simulink model "EPD_5_gen_with_limits_dell_p_values"  (R2021b)
settings: Solver=VariableStepAuto  StartTime=0.0  StopTime=50  RelTol=1e-3
settings Model: Creator=vijay  LastModifiedBy=vijay

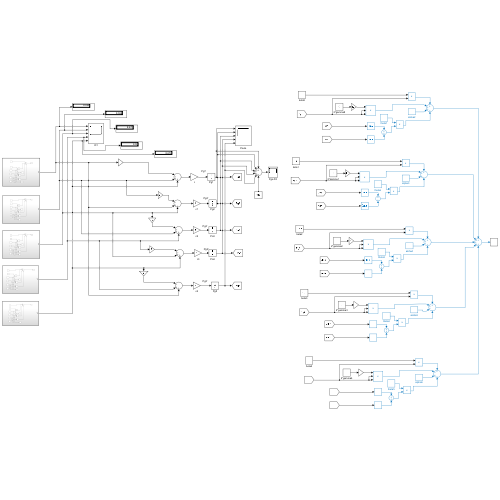
[thumbnail: Simulink's stored preview of the top-level diagram]
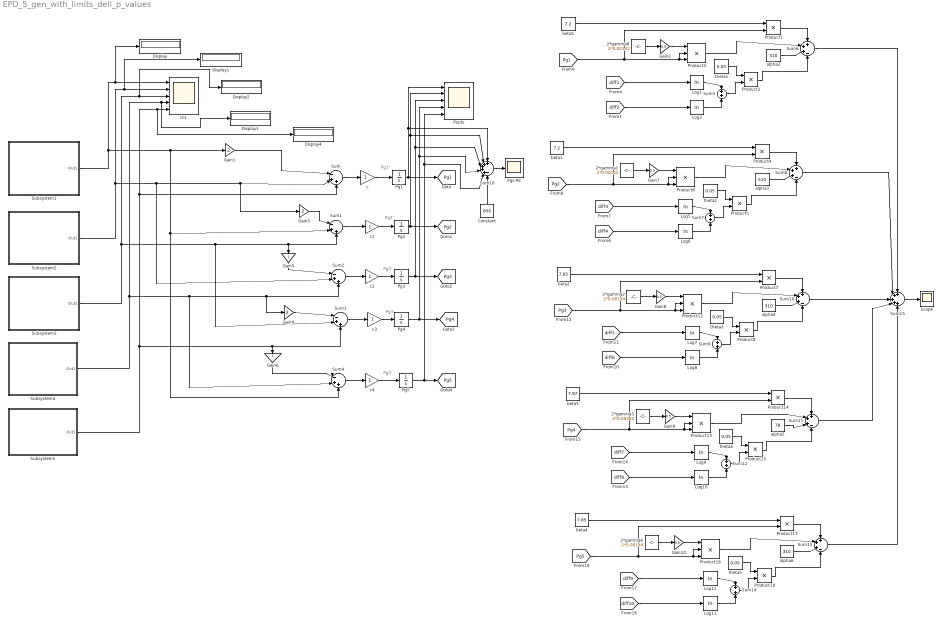
== system EPD_5_gen_with_limits_dell_p_values ==
  note: Pg3'
  note: Pg2'
  note: Pg1'
  note: Pg3'
  note: Pg3'
  2*gamma1 : Constant  Value=2*0.00142
  2*gamma2 : Constant  Value=2*0.00194
  2*gamma3 : Constant  Value=2*0.00482
  2*gamma4 : Constant  Value=2*0.00194
  2*gamma8 : Constant  Value=2*0.00142
  Constant : Constant  Value=850
  Display{,1..4} (5 alike) : Display
  Gain{1,3..6} (5 alike) : Gain  Gain=2
  Gain{2,7..10} (5 alike) : Gain  Gain=0.5
  IC1 : Scope  NumInputPorts=5
  Log{1,3,5..12} (10 alike) : Math  Operator=log  SignedPower=on  SaturateOnIntegerOverflow=on
  Pg1 : Integrator  InitialCondition=260
  Pg2 : Integrator  InitialCondition=260
  Pg3 : Integrator  InitialCondition=220
  Pg4 : Integrator  InitialCondition=170
  Pg5 : Integrator  InitialCondition=220
  Pgs-Pd : Scope
  Pouts : Scope  NumInputPorts=5
  Product{1..2,4..5,7..8,14..15,17..18} (10 alike) : Product
  Product{3,6,12..13,16} (5 alike) : Product  Inputs=3
  Scope : Scope
  Subsystem1 : Subsystem
  Subsystem2 : Subsystem
  Subsystem3 : Subsystem
  Subsystem4 : Subsystem
  Subsystem5 : Subsystem
  Sum{,1..4} (5 alike) : Sum  Inputs=|-++
  Sum{6,8,10..11,13} (5 alike) : Sum  Inputs=+++-
  Sum{5,7,9,12,14} (5 alike) : Sum
  Sum15 : Sum  Inputs=+++++
  Sum16 : Sum  Inputs=+++++-
  alpha2 : Constant  Value=510
  alpha3 : Constant  Value=510
  alpha4 : Constant  Value=310
  alpha5 : Constant  Value=78
  alpha6 : Constant  Value=310
  beta1 : Constant  Value=7.2
  beta2 : Constant  Value=7.85
  beta3 : Constant  Value=7.97
  beta4 : Constant  Value=7.85
  beta5 : Constant  Value=7.2
  c{,1..4} (5 alike) : Gain
  theta{1..5} (5 alike) : Constant  Value=0.05
  tag scope: Pg1=global, Pg2=global, Pg3=global, Pg4=global, Pg5=global
  wires:
  Subsystem1/1(Out1) -> Sum1/2, Sum4/3, Gain1/1, Display/1, IC1/1
  c/1 -> Pg1/1
  Sum2/1 -> c2/1
  Sum/1 -> c/1
  Pg3/1 -> Pouts/3, Sum16/3, [Pg3]
  Sum1/1 -> c1/1
  Pg2/1 -> [Pg2], Sum16/2, Pouts/2
  c1/1 -> Pg2/1
  c2/1 -> Pg3/1
  Pg1/1 -> Sum16/1, Pouts/1, [Pg1]
  c3/1 -> Pg4/1
  Pg4/1 -> Sum16/4, Pouts/4, [Pg4]
  Sum3/1 -> c3/1
  Sum4/1 -> c4/1
  Pg5/1 -> Sum16/5, Pouts/5, [Pg5]
  c4/1 -> Pg5/1
  Gain3/1 -> Sum1/1
  Subsystem2/1(Out1) -> Sum2/2, Gain3/1, Sum/2, Display1/1, IC1/2
  Subsystem3/1(Out1) -> Sum3/2, Gain5/1, Sum1/3, Display2/1, IC1/3
  Subsystem4/1(Out1) -> Sum4/2, Gain4/1, Sum2/3, Display3/1, IC1/4
  Subsystem5/1(Out1) -> Gain6/1, Sum3/3, Sum/3, Display4/1, IC1/5
  Gain1/1 -> Sum/1
  Gain5/1 -> Sum2/1
  Gain4/1 -> Sum3/1
  Gain6/1 -> Sum4/1
  2*gamma8/1 -> Gain2/1
  Product3/1 -> Sum6/2
  [Pg1] -> Product1/2, Product3/2, Product3/3
  [diff1] -> Log1/1
  Log1/1 -> Sum5/1
  Product2/1 -> Sum6/4
  Sum5/1 -> Product2/2
  Product1/1 -> Sum6/1
  alpha2/1 -> Sum6/3
  Log3/1 -> Sum5/2
  theta1/1 -> Product2/1
  beta5/1 -> Product1/1
  Gain2/1 -> Product3/1
  [diff2] -> Log3/1
  [diff4] -> Log6/1
  Gain7/1 -> Product6/1
  beta1/1 -> Product4/1
  theta2/1 -> Product5/1
  Log6/1 -> Sum7/2
  alpha3/1 -> Sum8/3
  Product4/1 -> Sum8/1
  Sum7/1 -> Product5/2
  Product5/1 -> Sum8/4
  Log5/1 -> Sum7/1
  [diff3] -> Log5/1
  [Pg2] -> Product6/3, Product6/2, Product4/2
  Product6/1 -> Sum8/2
  2*gamma1/1 -> Gain7/1
  2*gamma2/1 -> Gain8/1
  Product12/1 -> Sum10/2
  [Pg3] -> Product7/2, Product12/2, Product12/3
  [diff5] -> Log7/1
  Log7/1 -> Sum9/1
  Product8/1 -> Sum10/4
  Sum9/1 -> Product8/2
  Product7/1 -> Sum10/1
  alpha4/1 -> Sum10/3
  Log8/1 -> Sum9/2
  theta3/1 -> Product8/1
  beta2/1 -> Product7/1
  Gain8/1 -> Product12/1
  [diff6] -> Log8/1
  [diff8] -> Log10/1
  Gain9/1 -> Product13/1
  beta3/1 -> Product14/1
  theta4/1 -> Product15/1
  Log10/1 -> Sum12/2
  alpha5/1 -> Sum11/3
  Product14/1 -> Sum11/1
  Sum12/1 -> Product15/2
  Product15/1 -> Sum11/4
  Log9/1 -> Sum12/1
  [diff7] -> Log9/1
  [Pg4] -> Product13/3, Product13/2, Product14/2
  Product13/1 -> Sum11/2
  2*gamma3/1 -> Gain9/1
  2*gamma4/1 -> Gain10/1
  Product16/1 -> Sum13/2
  [Pg5] -> Product17/2, Product16/2, Product16/3
  [diff9] -> Log12/1
  Log12/1 -> Sum14/1
  Product18/1 -> Sum13/4
  Sum14/1 -> Product18/2
  Product17/1 -> Sum13/1
  alpha6/1 -> Sum13/3
  Log11/1 -> Sum14/2
  theta5/1 -> Product18/1
  beta4/1 -> Product17/1
  Gain10/1 -> Product16/1
  [diff10] -> Log11/1
  Sum6/1 -> Sum15/1
  Sum8/1 -> Sum15/2
  Sum10/1 -> Sum15/3
  Sum11/1 -> Sum15/4
  Sum13/1 -> Sum15/5
  Sum15/1 -> Scope/1
  Constant/1 -> Sum16/6
  Sum16/1 -> Pgs-Pd/1

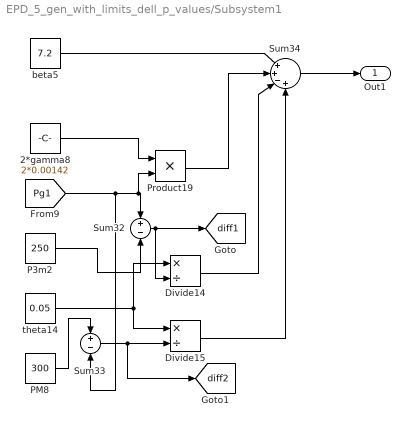
== system EPD_5_gen_with_limits_dell_p_values/Subsystem1 ==
  2*gamma8 : Constant  Value=2*0.00142
  Divide14 : Product  Inputs=*/
  Divide15 : Product  Inputs=*/
  P3m2 : Constant  Value=250
  PM8 : Constant  Value=300
  Product19 : Product
  Sum32 : Sum  Inputs=+-
  Sum33 : Sum  Inputs=+-
  Sum34 : Sum  Inputs=|++-+
  beta5 : Constant  Value=7.2
  theta14 : Constant  Value=0.05
  Out1 : Outport
  tag scope: diff1=global, diff2=global
  wires:
  Sum34/1 -> Out1/1
  2*gamma8/1 -> Product19/1
  Divide14/1 -> Sum34/3
  Divide15/1 -> Sum34/4
  PM8/1 -> Sum33/1
  [Pg1] -> Product19/2, Sum32/1, Sum33/2
  beta5/1 -> Sum34/1
  theta14/1 -> Divide14/1, Divide15/1
  Product19/1 -> Sum34/2
  Sum32/1 -> [diff1], Divide14/2
  P3m2/1 -> Sum32/2
  Sum33/1 -> [diff2], Divide15/2

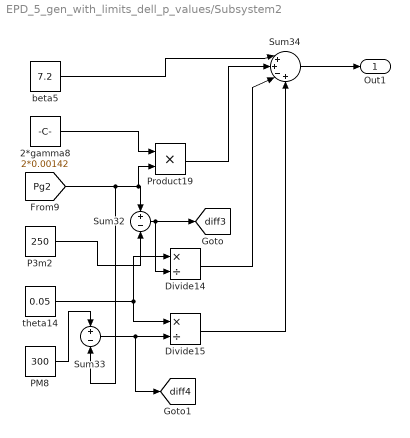
== system EPD_5_gen_with_limits_dell_p_values/Subsystem2 ==
  2*gamma8 : Constant  Value=2*0.00142
  Divide14 : Product  Inputs=*/
  Divide15 : Product  Inputs=*/
  P3m2 : Constant  Value=250
  PM8 : Constant  Value=300
  Product19 : Product
  Sum32 : Sum  Inputs=+-
  Sum33 : Sum  Inputs=+-
  Sum34 : Sum  Inputs=|++-+
  beta5 : Constant  Value=7.2
  theta14 : Constant  Value=0.05
  Out1 : Outport
  tag scope: diff3=global, diff4=global
  wires:
  Sum33/1 -> [diff4], Divide15/2
  P3m2/1 -> Sum32/2
  Sum32/1 -> [diff3], Divide14/2
  Product19/1 -> Sum34/2
  theta14/1 -> Divide15/1, Divide14/1
  beta5/1 -> Sum34/1
  [Pg2] -> Sum33/2, Sum32/1, Product19/2
  PM8/1 -> Sum33/1
  Divide15/1 -> Sum34/4
  Divide14/1 -> Sum34/3
  2*gamma8/1 -> Product19/1
  Sum34/1 -> Out1/1

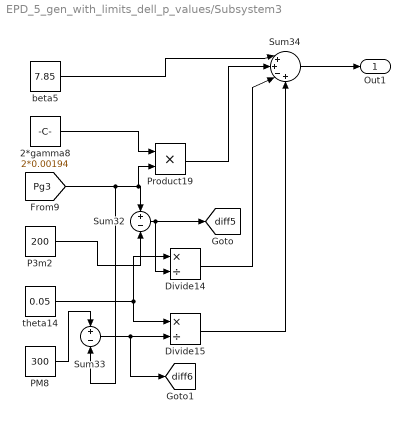
== system EPD_5_gen_with_limits_dell_p_values/Subsystem3 ==
  2*gamma8 : Constant  Value=2*0.00194
  Divide14 : Product  Inputs=*/
  Divide15 : Product  Inputs=*/
  P3m2 : Constant  Value=200
  PM8 : Constant  Value=300
  Product19 : Product
  Sum32 : Sum  Inputs=+-
  Sum33 : Sum  Inputs=+-
  Sum34 : Sum  Inputs=|++-+
  beta5 : Constant  Value=7.85
  theta14 : Constant  Value=0.05
  Out1 : Outport
  tag scope: diff5=global, diff6=global
  wires:
  Sum34/1 -> Out1/1
  2*gamma8/1 -> Product19/1
  Divide14/1 -> Sum34/3
  Divide15/1 -> Sum34/4
  PM8/1 -> Sum33/1
  [Pg3] -> Product19/2, Sum32/1, Sum33/2
  beta5/1 -> Sum34/1
  theta14/1 -> Divide14/1, Divide15/1
  Product19/1 -> Sum34/2
  Sum32/1 -> [diff5], Divide14/2
  P3m2/1 -> Sum32/2
  Sum33/1 -> [diff6], Divide15/2

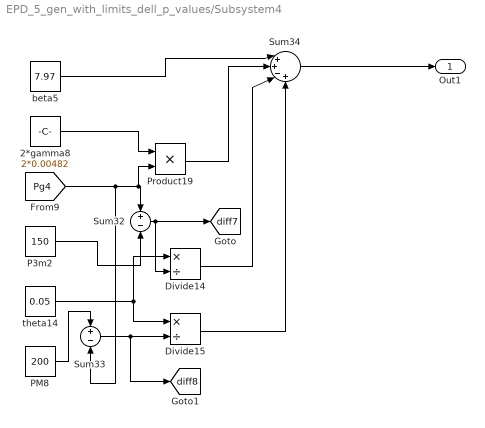
== system EPD_5_gen_with_limits_dell_p_values/Subsystem4 ==
  2*gamma8 : Constant  Value=2*0.00482
  Divide14 : Product  Inputs=*/
  Divide15 : Product  Inputs=*/
  P3m2 : Constant  Value=150
  PM8 : Constant  Value=200
  Product19 : Product
  Sum32 : Sum  Inputs=+-
  Sum33 : Sum  Inputs=+-
  Sum34 : Sum  Inputs=|++-+
  beta5 : Constant  Value=7.97
  theta14 : Constant  Value=0.05
  Out1 : Outport
  tag scope: diff7=global, diff8=global
  wires:
  Sum34/1 -> Out1/1
  [Pg4] -> Product19/2, Sum32/1, Sum33/2
  Product19/1 -> Sum34/2
  PM8/1 -> Sum33/1
  Divide15/1 -> Sum34/4
  Divide14/1 -> Sum34/3
  2*gamma8/1 -> Product19/1
  Sum33/1 -> [diff8], Divide15/2
  Sum32/1 -> [diff7], Divide14/2
  beta5/1 -> Sum34/1
  P3m2/1 -> Sum32/2
  theta14/1 -> Divide14/1, Divide15/1

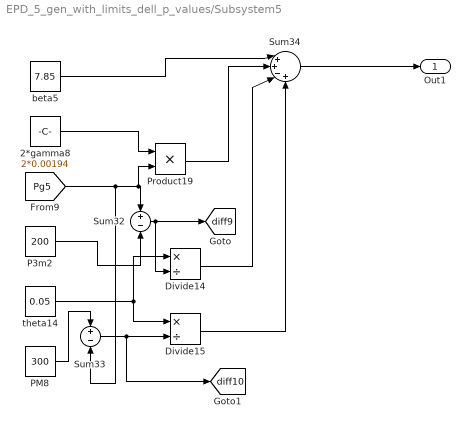
== system EPD_5_gen_with_limits_dell_p_values/Subsystem5 ==
  2*gamma8 : Constant  Value=2*0.00194
  Divide14 : Product  Inputs=*/
  Divide15 : Product  Inputs=*/
  P3m2 : Constant  Value=200
  PM8 : Constant  Value=300
  Product19 : Product
  Sum32 : Sum  Inputs=+-
  Sum33 : Sum  Inputs=+-
  Sum34 : Sum  Inputs=|++-+
  beta5 : Constant  Value=7.85
  theta14 : Constant  Value=0.05
  Out1 : Outport
  tag scope: diff10=global, diff9=global
  wires:
  Sum34/1 -> Out1/1
  [Pg5] -> Product19/2, Sum32/1, Sum33/2
  Product19/1 -> Sum34/2
  PM8/1 -> Sum33/1
  Divide15/1 -> Sum34/4
  Divide14/1 -> Sum34/3
  2*gamma8/1 -> Product19/1
  Sum33/1 -> [diff10], Divide15/2
  Sum32/1 -> [diff9], Divide14/2
  beta5/1 -> Sum34/1
  P3m2/1 -> Sum32/2
  theta14/1 -> Divide14/1, Divide15/1
